simulink model "StateFlowSimulink"  (R2021a)
settings: Solver=FixedStepDiscrete  StartTime=0.0  StopTime=inf  FixedStep=0.1  RelTol=1e-3  EnableMultiTasking=on
settings Model: SimulationMode=accelerator  Creator=Bishoy  LastModifiedBy=Bishoy
settings SolverCC: AlgebraicLoopSolver=TrustRegion  AutoInsertRateTranBlk=on
settings DataIOCC: LimitDataPoints=on
settings OptimizationCC: LifeSpan=inf
settings DebuggingCC: AllowSymbolicDim=off  SFUnexpectedBacktrackingDiag=warning  SFNoUnconditionalDefaultTransitionDiag=warning  SFExecutionAtInitializationDiag=none  ArithmeticOperatorsInVariantConditions=warning
settings SFSimCC: SimUseLocalCustomCode=off  CustomCodeUndefinedFunction=UseInterfaceOnly
settings RTWCC: RTWUseLocalCustomCode=off
settings CodeAppCC: StateflowObjectComments=on
settings GRTTargetCC: TargetLangStandard=C89/C90 (ANSI)
settings ConfigComp: CovMetricSettings=dw  CovSaveCumulativeToWorkspaceVar=on  CovSaveSingleToWorkspaceVar=on  CovExternalEMLEnable=off  CovSFcnEnable=off

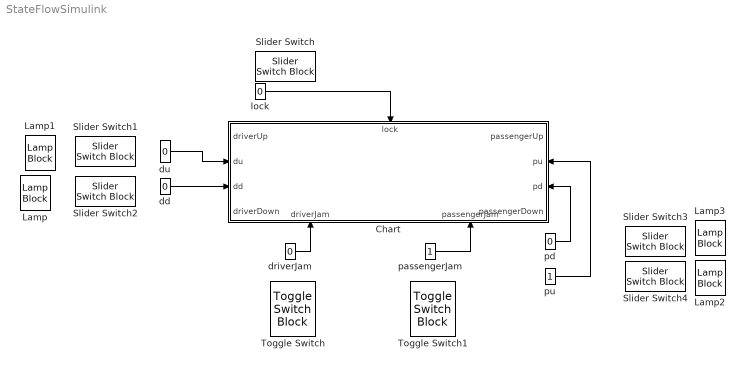
== system StateFlowSimulink ==
  Chart : Stateflow chart  TreatAsAtomicUnit=on
      settings: PortSchema="{\"entries\":[{\"content\":{\"sides\":[{\"content\":{\"connectorIds\":[\"Out2\",\"In2\",\"In1\",\"Out1\"]},\"type\":\"ConnectorPlacement.EquallySpacedRectSide\",\"uuid\":\"b9ec05ff-a259-487f-9204-6d6e9e59d55e\"},{\"content\":{\"connectorIds\":[\"Out4\",\"In4\",\"In3\",\"Out3\"],\"side\":\"RIGHT\"},\"type\":\"ConnectorPlacement.EquallySpacedRectSide\",\"uuid\":\"a8e100df-298e-4c1e-8458-4d2f07c6803f\"},{\"content\":{\"connectorIds\":[\"In5\"],\"side\":\"TOP\"},\"type\":\"ConnectorPlacement.EquallySpacedRectSide\",\"uuid\":\"3c7e78eb-d52f-4ead-8297-87dfc1a95edc\"},{\"content\":{\"connectorIds\":[\"In6\",\"In7\"],\"side\":\"BOTTOM\"},\"type\":\"ConnectorPlacement.EquallySpacedRectSide\",\"uuid\":\"273cb3cb-a5bb-4704-8fd8-a6bfbbe6e702\"}]},\"type\":\"ConnectorPlacement.EquallySpacedConnector\",\"uuid\":\"ef133a53-f3a1-472e-9bf4-7738adb61131\"}],\"packageUris\":[\"http://schema.mathworks.com/mf0/Connector/R2020b\"],\"version\":\"1.0\"}"
  Lamp{,1..3} (4 alike) : LampBlock
  Slider Switch{,1..4} (5 alike) : SliderSwitchBlock
      settings: Values={{'Off', 'On'}, [0 1]}
  Toggle Switch : ToggleSwitchBlock
      settings: Values={{'Off', 'On'}, [0 1]}
  Toggle Switch1 : ToggleSwitchBlock
      settings: Values={{'Off', 'On'}, [0 1]}
  dd : Constant  Value=0
  driverJam : Constant  Value=0
  du : Constant  Value=0
  lock : Constant  Value=0
  passengerJam : Constant
  pd : Constant  Value=0
  pu : Constant
  wires:
  dd/1 -> Chart/1(dd)
  du/1 -> Chart/2(du)
  pu/1 -> Chart/4(pu)
  pd/1 -> Chart/3(pd)
  lock/1 -> Chart/5(lock)
  driverJam/1 -> Chart/6(driverJam)
  passengerJam/1 -> Chart/7(passengerJam)

== stateflow chart StateFlowSimulink/Chart ==
  state driverEmergencyDown
    entry:
    driverDown=1;
    driverUp=0;
  state passengerEmergencyDown
    entry:
    passengerDown=1;
    passengerUp=0;
  state driverOff
    entry:
    driverUp=0;
    driverDown=0;
  state passengerOff
    entry:
    passengerDown=0;
    passengerUp=0;
  state passengerUp
    entry:
    passengerUp=1;
    passengerDown=0;
    state initPassengerUp
    state autoPassengerUp
    state manualPassengerUp
    (default) -> initPassengerUp
    initPassengerUp -> (junction 134) : after(100, tick)
    (junction 134) -> autoPassengerUp [order 1] : [~pu]
    (junction 134) -> manualPassengerUp [order 2]
  state passengerDown
    entry:
    passengerUp=0;
    passengerDown=1;
    state initPassengerDown
    state autoDriverDown
    state manualDriverDown
    (default) -> initPassengerDown
    initPassengerDown -> (junction 143) : after(100, tick)
    (junction 143) -> passengerDown.autoDriverDown [order 1] : [~pd]
    (junction 143) -> passengerDown.manualDriverDown [order 2]
  state driverUp
    entry:
    driverUp=1;
    driverDown=0;
    state initDriverUp
    state autoDriverUp
    state manualDriverUp
    (default) -> initDriverUp
    initDriverUp -> (junction 115) : after(100, tick)
    (junction 115) -> autoDriverUp [order 1] : [~du]
    (junction 115) -> manualDriverUp [order 2]
  state driverDown
    entry:
    driverDown = 1;
    driverUp = 0;
    state initDriverDown
    state autoDriverDown
    state manualDriverDown
    (default) -> initDriverDown
    initDriverDown -> (junction 107) : after(100, tick)
    (junction 107) -> driverDown.autoDriverDown [order 1] : [~dd]
    (junction 107) -> driverDown.manualDriverDown [order 2]
  (default) -> passengerOff
  passengerEmergencyDown -> passengerOff : after(0.5, sec)
  driverEmergencyDown -> driverOff : after(0.5, sec)
  driverDown.autoDriverDown -> driverOff : after(5, sec)
  driverUp -> driverEmergencyDown : [driverJam]
  autoPassengerUp -> passengerOff : after(5, sec)
  passengerDown.manualDriverDown -> passengerOff : [~pd || lock]
  passengerUp -> passengerEmergencyDown : [passengerJam]
  manualDriverUp -> driverOff : [~du]
  driverDown.manualDriverDown -> driverOff : [~dd]
  driverOff -> driverDown [order 2] : [dd]
  autoDriverUp -> driverOff : after(5, sec)
  driverOff -> driverUp [order 1] : [du]
  passengerOff -> passengerUp [order 1] : [pu && ~lock]
  manualPassengerUp -> passengerOff : [~pu || lock]
  passengerDown.autoDriverDown -> passengerOff : after(5, sec)
  passengerOff -> passengerDown [order 2] : [pd && ~lock]
  data: dd input; du input; pd input; pu input; lock input; driverDown output; driverUp output; passengerDown output; passengerUp output; driverJam input; passengerJam input
